simulink model "WMR_ROS_MATMPC_SIMULINK_real"  (R2022b)
settings: Solver=FixedStepAuto  StartTime=0.0  StopTime=100  FixedStep=0.02  RelTol=1e-3
model workspace (MAT data in the model file):
  SL_ROS_VariableLengthArrays_MaxSizes.CommonInfo.ArrayTruncateAction = 'EmitWarning'
  SL_ROS_VariableLengthArrays_MaxSizes.MsgTypeMap = containers.Map
  SL_ROS_VariableLengthArrays_MaxSizes.MsgTypeMap.serialization.keys = {'nav_msgs/OccupancyGrid'}
  SL_ROS_VariableLengthArrays_MaxSizes.MsgTypeMap.serialization.values{1}.PropertyName = 'Data'
  SL_ROS_VariableLengthArrays_MaxSizes.MsgTypeMap.serialization.values{1}.DataType = 'int8'
  SL_ROS_VariableLengthArrays_MaxSizes.MsgTypeMap.serialization.values{1}.MaxLength = 40000
  SL_ROS_VariableLengthArrays_MaxSizes.MsgTypeMap.serialization.uniformity = 0
  SL_ROS_VariableLengthArrays_MaxSizes.MsgTypeMap.serialization.keyType = 'char'
  SL_ROS_VariableLengthArrays_MaxSizes.MsgTypeMap.serialization.valueType = 'any'
values from neighbouring files (symbols this model uses):
  costmap_resolution = 0.1    [Initialization_Simulink.m]
  costmap_width = 100    [Initialization_Simulink.m]
  lb = 0    [Initialization_Simulink.m]
  lb_x = [0;0]    [InitData.m]    (also in Initialization_Simulink.m = [0; -0.8])
  lbu = -inf(nu,1)    [InitData.m]    (also in Initialization_Simulink.m = repmat(lbu,1,N))
  lbx = 0    [Initialization_Simulink.m]
  N = settings.N    [InitData.m]    (also in InitMemory.m; Initialization_Simulink.m = 100; Simulation.m = 10)
  np = settings.np    [InitData.m]    (also in InitMemory.m; Initialization_Simulink.m; Simulation.m)
  Ts = settings.Ts_st    [Initialization_Simulink.m]    (also in Simulation.m)
  ub = 0    [Initialization_Simulink.m]
  ub_x = [100;100]    [InitData.m]    (also in Initialization_Simulink.m = [0.3; 0.8])
  ubu = inf(nu,1)    [InitData.m]    (also in Initialization_Simulink.m = repmat(ubu,1,N))
  ubx = 0    [Initialization_Simulink.m]
  W = repmat(w,1,N)    [Initialization_Simulink.m]
  WN = [50 50 0 50 50]'    [Initialization_Simulink.m]
  z0 = 0    [Initialization_Simulink.m]
undefined symbols (not defined in the file or in its folder): Angular, DiscIntNeverNeededParam, Linear, myref, opt, settings, X, X_SL_Info, Y, Y_SL_Info
libraries: robotlib x8, robotcorelib x2
settings Model: SimulationMode=accelerator  Creator=chen  LastModifiedBy=niccoloturcato
settings SolverCC: AlgebraicLoopSolver=TrustRegion
settings DataIOCC: SaveFormat=StructureWithTime
settings OptimizationCC: EnhancedBackFolding=on  PassReuseOutputArgsAs=Individual arguments  ZeroExternalMemoryAtStartup=off  ZeroInternalMemoryAtStartup=off  MaxStackSize=64  OptimizeBlockOrder=speed  DifferentSizesBufferReuse=on  OptimizationCustomize=off  EfficientTunableParamExpr=on
settings DebuggingCC: ParameterTunabilityLossMsg=error  UnconnectedInputMsg=warning  UnconnectedOutputMsg=warning  UnconnectedLineMsg=warning  SFMachineParentedDataDiag=warning  ArithmeticOperatorsInVariantConditions=warning
settings HardwareCC: ProdBitPerPointer=32  ProdBitPerSizeT=32  ProdBitPerPtrDiffT=32  ProdLargestAtomicFloat=None  ProdIntDivRoundTo=Undefined  ProdEndianess=Unspecified  ProdWordSize=32  ProdHWDeviceType=Generic->Unspecified (assume 32-bit Generic)  UseEmbeddedCoderFeatures=off
settings ModelReferenceCC: EnableRefExpFcnMdlSchedulingChecks=on
settings SFSimCC: SimUseLocalCustomCode=off  MATLABDynamicMemAlloc=off  CustomCodeUndefinedFunction=UseInterfaceOnly
settings RTWCC: Description=Embedded Coder  SystemTargetFile=ert.tlc  HardwareBoard=Robot Operating System (ROS)  TLCOptions="-aInlineSetEventsForThisBaseRateFcn=TLC_FALSE -aSuppressMultiTaskScheduler=TLC_FALSE  -aRateBasedStepFcn=0"  TemplateMakefile=ert_default_tmf  RTWUseLocalCustomCode=off  Toolchain=Catkin  TargetLang=C++  CheckMdlBeforeBuild=Error
settings CodeAppCC: ForceParamTrailComments=on  IgnoreCustomStorageClasses=off  OperatorAnnotations=on  SimulinkDataObjDesc=on  SFDataObjDesc=on  InsertBlockDesc=on
settings ERTTargetCC: SupportNonInlinedSFcns=on

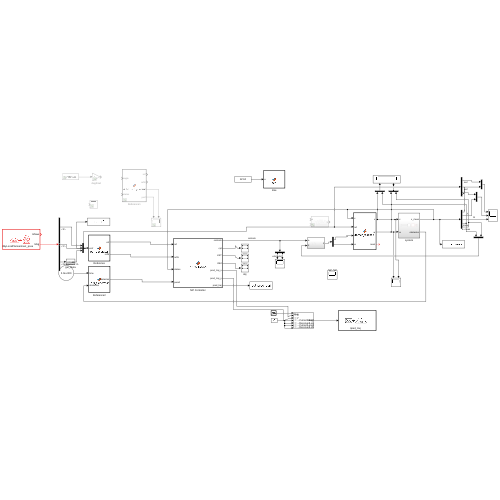
[thumbnail: Simulink's stored preview of the top-level diagram]
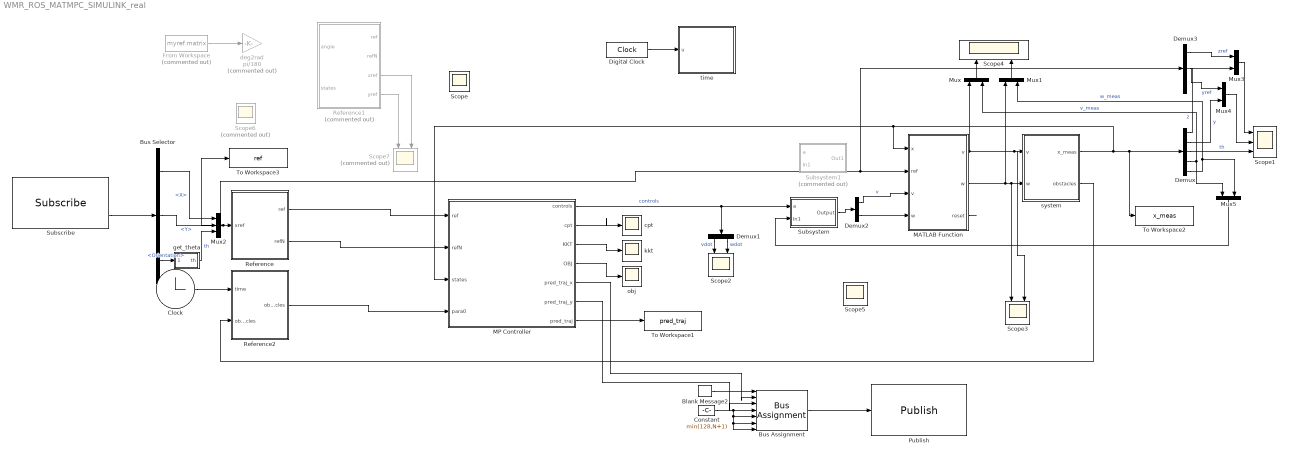
== system WMR_ROS_MATMPC_SIMULINK_real ==
  Blank Message2 : robotlib/Blank Message  messageClass=Message  entityType=wheelchair_iaslab_control/matArray  messageType=wheelchair_iaslab_control/matArray  SampleTime=-1  legacyBusStruct=off
  Bus Assignment : BusAssignment  AssignedSignals=X,Y,X_SL_Info.CurrentLength,X_SL_Info.ReceivedLength,Y_SL_Info.CurrentLength,Y_SL_Info.ReceivedLength
  Bus Selector : BusSelector  DialogController=Simulink.DDGSource_BusSelector  OutputSignals=Position.X,Position.Y,Orientation
  Clock : Clock
  Constant : Constant  Value=min(128,N+1)  OutDataTypeStr=uint32
  Demux : Demux  Outputs=5
  Demux1 : Demux  Outputs=2
  Demux2 : Demux  Outputs=2
  Demux3 : Demux  Outputs=3
  Digital Clock : DigitalClock  SampleTime=-1
  From Workspace : FromWorkspace  Commented=on  VariableName=myref.matrix  SampleTime=myref.T
  MATLAB Function : MATLAB Function  TreatAsAtomicUnit=on
  MP Controller : MATLAB Function  TreatAsAtomicUnit=on  SystemSampleTime=Ts
  Mux{,1,3..5} (5 alike) : Mux  Inputs=2
  Mux2 : Mux  Inputs=3
  Publish : robotlib/Publish  topicSource=Specify your own  topic=/pred_traj  messageType=wheelchair_iaslab_control/matArray  legacyBusStruct=off  messageQueueLength=1
      settings: LibrarySourceBlock=roslib/ROS/Publish
  Reference : MATLAB Function  TreatAsAtomicUnit=on
  Reference1 : MATLAB Function  Commented=on  TreatAsAtomicUnit=on
  Reference2 : MATLAB Function  TreatAsAtomicUnit=on
  Scope1 : Scope  NumInputPorts=3
  Scope{2..5} (4 alike) : Scope  NumInputPorts=2
  Scope6 : Scope  Commented=on
  Scope7 : Scope  Commented=on  NumInputPorts=2
  Subscribe : robotlib/Subscribe  topicSource=Specify your own  topic=/move_base/MyLocalPlanner/next_pose  messageType=geometry_msgs/Pose  SampleTime=0.2  legacyBusStruct=off  messageQueueLength=1
      settings: LibrarySourceBlock=roslib/ROS/Subscribe
  Subsystem : Subsystem
  Subsystem1 : Subsystem  Commented=on
  To Workspace1 : ToWorkspace  VariableName=pred_traj  SaveFormat=Structure With Time  SampleTime=-1
  To Workspace2 : ToWorkspace  VariableName=x_meas  SaveFormat=Structure With Time  SampleTime=-1
  To Workspace3 : ToWorkspace  VariableName=ref  SaveFormat=Structure With Time  SampleTime=-1
  cpt : Scope
  deg2rad : Gain  Commented=on  Gain=pi/180
  get_theta : Subsystem
  kkt : Scope
  obj : Scope
  system : Subsystem
  time : MATLAB Function  TreatAsAtomicUnit=on  SystemSampleTime=Ts
  Scope : Scope
  wires:
  MP Controller/1(controls) -> Subsystem/1(a), Demux1/1  "controls"
  MP Controller/2(cpt) -> cpt/1
  MP Controller/4(OBJ) -> obj/1
  MP Controller/3(KKT) -> kkt/1
  Demux/3 -> Scope1/3  "th"
  Demux/1 -> Mux3/2  "z"
  Demux/2 -> Mux4/2  "y"
  Demux/5 -> Mux5/2, Mux1/2  "w_meas"
  Demux/4 -> Mux/2, Mux5/1  "v_meas"
  Demux1/1 -> Scope2/1  "vdot"
  Demux1/2 -> Scope2/2  "wdot"
  Mux/1 -> Scope4/1
  Mux1/1 -> Scope4/2
  Blank Message2/1 -> Bus Assignment/1
  Bus Assignment/1 -> Publish/1
  MP Controller/6(pred_traj_y) -> Bus Assignment/3
  Constant/1 -> Bus Assignment/7, Bus Assignment/6, Bus Assignment/5, Bus Assignment/4
  Reference/1(ref) -> MP Controller/1(ref)
  Reference/2(refN) -> MP Controller/2(refN)
  From Workspace/1 -> deg2rad/1
  Reference1/3(zref) -> Scope7/2
  Reference1/4(yref) -> Scope7/1
  Clock/1 -> Reference2/1(time)
  Reference2/1(obstacles) -> MP Controller/4(para0)
  system/2(obstacles) -> Reference2/2("obstacles ")
  system/1(x_meas) -> To Workspace2/1, Demux/1, MP Controller/3(states), MATLAB Function/1(x)
  Subscribe/2 -> Bus Selector/1
  Bus Selector/1 -> Mux2/1  "<X>"
  Bus Selector/2 -> Mux2/2  "<Y>"
  Mux2/1 -> To Workspace3/1, Demux3/1, MATLAB Function/2(ref), Reference/1(xref)
  Demux2/1 -> MATLAB Function/3("v ")  "v"
  MATLAB Function/1(v) -> Scope3/2, system/1(v), Mux/1
  MATLAB Function/2(w) -> Scope3/1, system/2(w), Mux1/1
  MATLAB Function/3(reset) -> ?
  Demux3/1 -> Mux3/1  "zref"
  Mux3/1 -> Scope1/1
  Demux3/2 -> Mux4/1  "yref"
  Mux4/1 -> Scope1/2
  MP Controller/5(pred_traj_x) -> Bus Assignment/2
  MP Controller/7(pred_traj) -> To Workspace1/1
  Digital Clock/1 -> time/1(u)
  Bus Selector/3 -> get_theta/1(<Orientation>)  "<Orientation>"
  get_theta/1(th) -> Mux2/3  "th"
  Mux5/1 -> Subsystem/2(In1)
  Demux2/2 -> MATLAB Function/4("w ")
  Subsystem/1(Output) -> Demux2/1

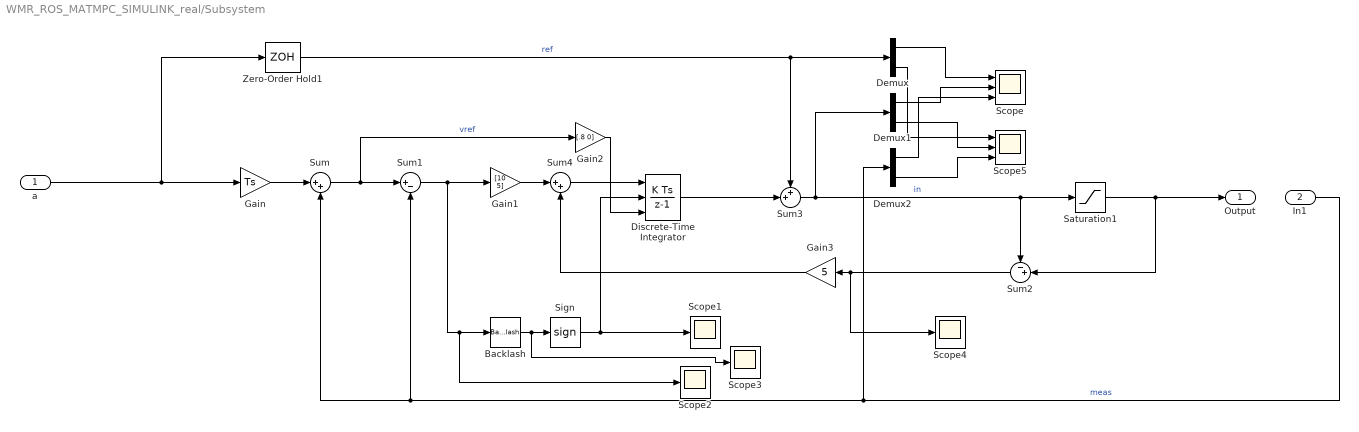
== system WMR_ROS_MATMPC_SIMULINK_real/Subsystem ==
  a : Inport
  In1 : Inport  Port=2
  Backlash : Backlash  BacklashWidth=0.01
  Demux : Demux  Outputs=2
  Demux1 : Demux  Outputs=2
  Demux2 : Demux  Outputs=2
  Discrete-Time Integrator : DiscreteIntegrator  ExternalReset=either  InitialConditionSource=external  SampleTime=-1  ICPrevOutput=DiscIntNeverNeededParam  ICPrevScaledInput=DiscIntNeverNeededParam
  Gain : Gain  Gain=Ts
  Gain1 : Gain  Gain=[10 5]
  Gain2 : Gain  Gain=[.8 0]
  Gain3 : Gain  Gain=5
  Saturation1 : Saturate  UpperLimit=ub_x  LowerLimit=[-0.1 lbx(2)]
  Scope : Scope  NumInputPorts=3
  Scope{1..4} (4 alike) : Scope
  Scope5 : Scope  NumInputPorts=3
  Sign : Signum
  Sum : Sum  Inputs=|++
  Sum1 : Sum  Inputs=|+-
  Sum2 : Sum  Inputs=-+|
  Sum3 : Sum  Inputs=++|
  Sum4 : Sum  Inputs=|++
  Zero-Order Hold1 : ZeroOrderHold  SampleTime=0.02
  Output : Outport
  wires:
  Gain/1 -> Sum/1
  Sum/1 -> Gain2/1, Sum1/1  "vref"
  Backlash/1 -> Scope3/1, Sign/1
  In1/1 -> Sum1/2, Sum/2, Demux2/1  "meas"
  Sum1/1 -> Scope2/1, Backlash/1, Gain1/1
  a/1 -> Zero-Order Hold1/1, Gain/1
  Zero-Order Hold1/1 -> Sum3/1, Demux/1  "ref"
  Discrete-Time Integrator/1 -> Sum3/2
  Sign/1 -> Scope1/1, Discrete-Time Integrator/2
  Gain2/1 -> Discrete-Time Integrator/3
  Sum3/1 -> Demux1/1, Saturation1/1, Sum2/1  "in"
  Saturation1/1 -> Output/1, Sum2/2
  Gain1/1 -> Sum4/1
  Sum4/1 -> Discrete-Time Integrator/1
  Gain3/1 -> Sum4/2
  Sum2/1 -> Scope4/1, Gain3/1
  Demux1/1 -> Scope/2
  Demux2/1 -> Scope/3
  Demux/1 -> Scope/1
  Demux/2 -> Scope5/1
  Demux1/2 -> Scope5/2
  Demux2/2 -> Scope5/3

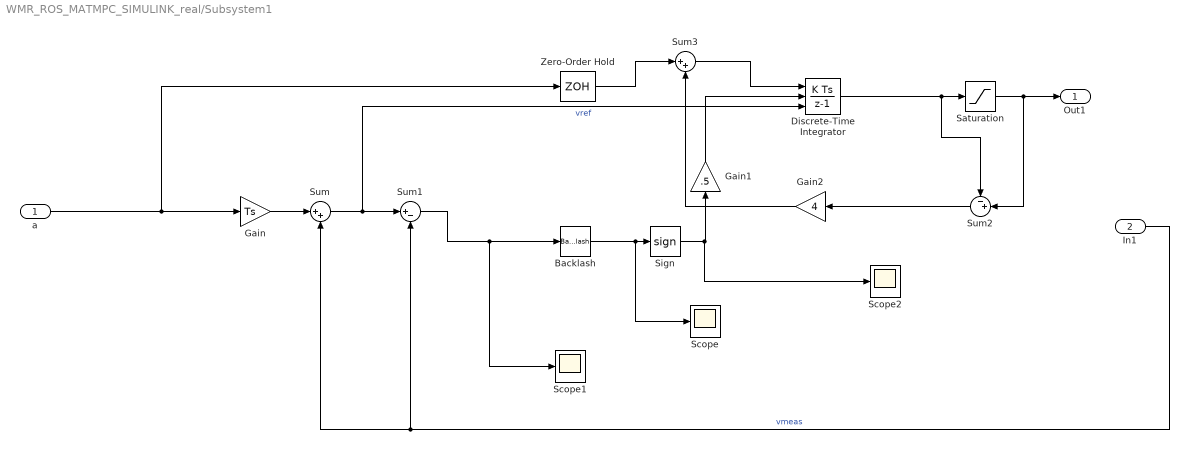
== system WMR_ROS_MATMPC_SIMULINK_real/Subsystem1 ==
  a : Inport
  In1 : Inport  Port=2
  Backlash : Backlash  BacklashWidth=0.01
  Discrete-Time Integrator : DiscreteIntegrator  ExternalReset=either  InitialConditionSource=external  SampleTime=-1  ICPrevOutput=DiscIntNeverNeededParam  ICPrevScaledInput=DiscIntNeverNeededParam
  Gain : Gain  Gain=Ts
  Gain1 : Gain  Gain=.5
  Gain2 : Gain  Gain=4
  Saturation : Saturate  UpperLimit=ub_x  LowerLimit=[-0.1 lbx(2)]
  Scope : Scope
  Scope1 : Scope
  Scope2 : Scope
  Sign : Signum
  Sum : Sum  Inputs=|++
  Sum1 : Sum  Inputs=|+-
  Sum2 : Sum  Inputs=-+|
  Sum3 : Sum  Inputs=|++
  Zero-Order Hold : ZeroOrderHold  SampleTime=0.02
  Out1 : Outport
  wires:
  Gain/1 -> Sum/1
  Sum/1 -> Discrete-Time Integrator/3, Sum1/1  "vref"
  Backlash/1 -> Scope/1, Sign/1
  In1/1 -> Sum1/2, Sum/2  "vmeas"
  Sum1/1 -> Scope1/1, Backlash/1
  Sign/1 -> Gain1/1, Scope2/1
  Discrete-Time Integrator/1 -> Sum2/1, Saturation/1
  Gain1/1 -> Discrete-Time Integrator/2
  Saturation/1 -> Sum2/2, Out1/1
  a/1 -> Zero-Order Hold/1, Gain/1
  Zero-Order Hold/1 -> Sum3/1
  Sum2/1 -> Gain2/1
  Gain2/1 -> Sum3/2
  Sum3/1 -> Discrete-Time Integrator/1

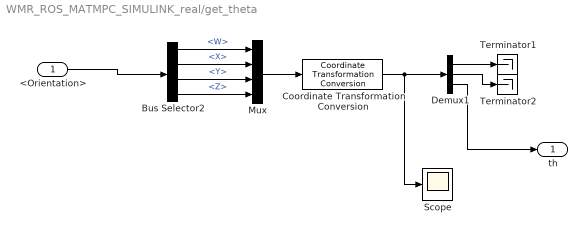
== system WMR_ROS_MATMPC_SIMULINK_real/get_theta ==
  <Orientation> : Inport
  Bus Selector2 : BusSelector  DialogController=Simulink.DDGSource_BusSelector  OutputSignals=W,X,Y,Z
  Coordinate Transformation Conversion : robotcorelib/Coordinate Transformation Conversion  InputRepresentation=Quaternion  InputEulerSequence=ZYX  ShowTrVecInputPort=on  OutputRepresentation=Euler Angles  OutputEulerSequence=XYZ  ShowTrVecOutputPort=on  SimulateUsing=Interpreted execution
      settings: LibrarySourceBlock=roslib/Utilities/Coordinate Transformation Conversion
  Demux1 : Demux  Outputs=3
  Mux : Mux
  Scope : Scope
  Terminator1 : Terminator
  Terminator2 : Terminator
  th : Outport
  wires:
  Bus Selector2/3 -> Mux/3  "<Y>"
  Demux1/1 -> Terminator1/1
  Bus Selector2/4 -> Mux/4  "<Z>"
  Bus Selector2/1 -> Mux/1  "<W>"
  Coordinate Transformation Conversion/1 -> Scope/1, Demux1/1
  <Orientation>/1 -> Bus Selector2/1
  Demux1/2 -> Terminator2/1
  Bus Selector2/2 -> Mux/2  "<X>"
  Mux/1 -> Coordinate Transformation Conversion/1
  Demux1/3 -> th/1

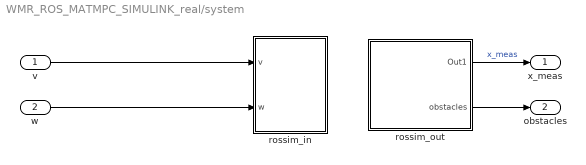
== system WMR_ROS_MATMPC_SIMULINK_real/system ==
  v : Inport
  w : Inport  Port=2
  rossim_in : Subsystem
  rossim_out : Subsystem
  x_meas : Outport
  obstacles : Outport  Port=2
  wires:
  w/1 -> rossim_in/2(w)
  v/1 -> rossim_in/1(v)
  rossim_out/1(Out1) -> x_meas/1  "x_meas"
  rossim_out/2(obstacles) -> obstacles/1

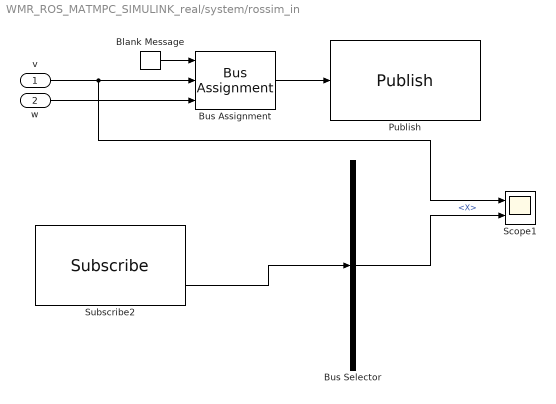
== system WMR_ROS_MATMPC_SIMULINK_real/system/rossim_in ==
  v : Inport
  w : Inport  Port=2
  Blank Message : robotlib/Blank Message  messageClass=Message  entityType=geometry_msgs/Twist  messageType=geometry_msgs/Twist  SampleTime=-1  legacyBusStruct=off
  Bus Assignment : BusAssignment  AssignedSignals=Linear.X,Angular.Z
  Bus Selector : BusSelector  DialogController=Simulink.DDGSource_BusSelector  OutputSignals=Linear.X
  Publish : robotlib/Publish  topicSource=Specify your own  topic=/cmd_vel  messageType=geometry_msgs/Twist  legacyBusStruct=off  messageQueueLength=1
      settings: LibrarySourceBlock=roslib/ROS/Publish
  Scope1 : Scope  NumInputPorts=2
  Subscribe2 : robotlib/Subscribe  topicSource=Specify your own  topic=/cmd_vel  messageType=geometry_msgs/Twist  SampleTime=0.020  legacyBusStruct=off  messageQueueLength=1
      settings: LibrarySourceBlock=roslib/ROS/Subscribe
  wires:
  Blank Message/1 -> Bus Assignment/1
  Bus Assignment/1 -> Publish/1
  v/1 -> Scope1/1, Bus Assignment/2
  Subscribe2/2 -> Bus Selector/1
  Bus Selector/1 -> Scope1/2  "<X>"
  w/1 -> Bus Assignment/3

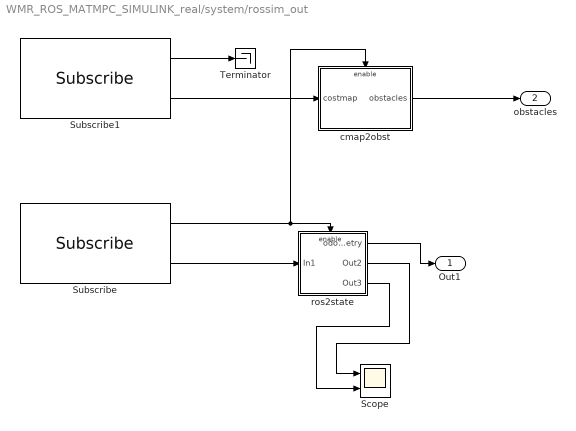
== system WMR_ROS_MATMPC_SIMULINK_real/system/rossim_out ==
  Scope : Scope  NumInputPorts=2
  Subscribe : robotlib/Subscribe  topicSource=Specify your own  topic=/odom  messageType=nav_msgs/Odometry  SampleTime=0.020  legacyBusStruct=off  messageQueueLength=1
      settings: LibrarySourceBlock=roslib/ROS/Subscribe
  Subscribe1 : robotlib/Subscribe  topicSource=Select from ROS network  topic=/move_base/local_costmap/costmap  messageType=nav_msgs/OccupancyGrid  SampleTime=0.02  legacyBusStruct=off  messageQueueLength=1
      settings: LibrarySourceBlock=roslib/ROS/Subscribe
  Terminator : Terminator
  cmap2obst : Subsystem
  ros2state : Subsystem
  Out1 : Outport
  obstacles : Outport  Port=2
  wires:
  Subscribe/1 -> ros2state/Enable, cmap2obst/Enable
  Subscribe/2 -> ros2state/1(In1)
  ros2state/1(odometry) -> Out1/1
  ros2state/2(Out2) -> Scope/1
  ros2state/3(Out3) -> Scope/2
  Subscribe1/1 -> Terminator/1
  Subscribe1/2 -> cmap2obst/1(costmap)
  cmap2obst/1(obstacles) -> obstacles/1

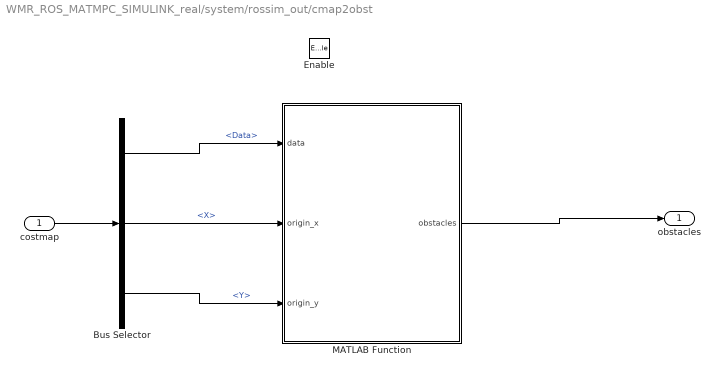
== system WMR_ROS_MATMPC_SIMULINK_real/system/rossim_out/cmap2obst ==
  costmap : Inport
  Enable : EnablePort  StatesWhenEnabling=reset
  Bus Selector : BusSelector  DialogController=Simulink.DDGSource_BusSelector  OutputSignals=Data,Info.Origin.Position.X,Info.Origin.Position.Y
  MATLAB Function : MATLAB Function  TreatAsAtomicUnit=on
  obstacles : Outport
  wires:
  costmap/1 -> Bus Selector/1
  MATLAB Function/1(obstacles) -> obstacles/1
  Bus Selector/3 -> MATLAB Function/3(origin_y)  "<Y>"
  Bus Selector/2 -> MATLAB Function/2(origin_x)  "<X>"
  Bus Selector/1 -> MATLAB Function/1(data)  "<Data>"

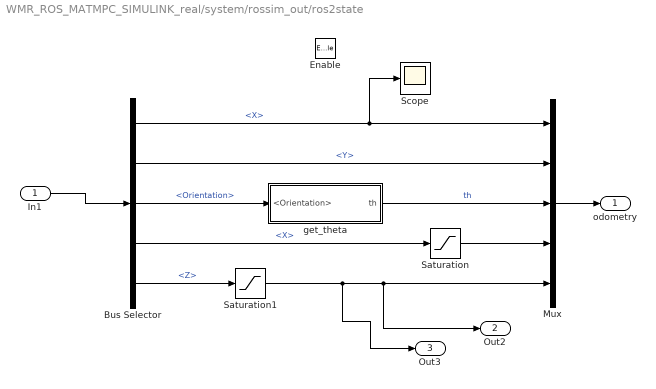
== system WMR_ROS_MATMPC_SIMULINK_real/system/rossim_out/ros2state ==
  In1 : Inport
  Enable : EnablePort  StatesWhenEnabling=reset
  Bus Selector : BusSelector  DialogController=Simulink.DDGSource_BusSelector  OutputSignals=Pose.Pose.Position.X,Pose.Pose.Position.Y,Pose.Pose.Orientation,Twist.Twist.Linear.X,Twist.Twist.Angular.Z
  Mux : Mux  Inputs=5
  Saturation : Saturate  UpperLimit=ub_x(1)  LowerLimit=lb_x(1)
  Saturation1 : Saturate  UpperLimit=ub_x(2)  LowerLimit=lb_x(2)
  Scope : Scope
  get_theta : Subsystem
  odometry : Outport
  Out2 : Outport  Port=2
  Out3 : Outport  Port=3
  wires:
  Bus Selector/5 -> Saturation1/1  "<Z>"
  Bus Selector/1 -> Mux/1, Scope/1  "<X>"
  In1/1 -> Bus Selector/1
  get_theta/1(th) -> Mux/3  "th"
  Bus Selector/2 -> Mux/2  "<Y>"
  Bus Selector/3 -> get_theta/1(<Orientation>)  "<Orientation>"
  Bus Selector/4 -> Saturation/1  "<X>"
  Mux/1 -> odometry/1
  Saturation/1 -> Mux/4
  Saturation1/1 -> Mux/5, Out2/1, Out3/1

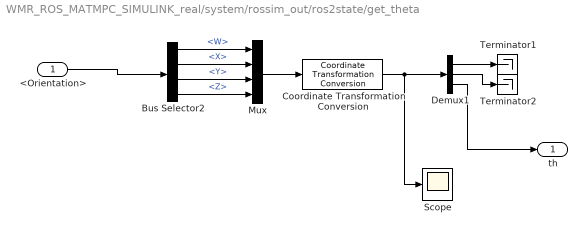
== system WMR_ROS_MATMPC_SIMULINK_real/system/rossim_out/ros2state/get_theta ==
  <Orientation> : Inport
  Bus Selector2 : BusSelector  DialogController=Simulink.DDGSource_BusSelector  OutputSignals=W,X,Y,Z
  Coordinate Transformation Conversion : robotcorelib/Coordinate Transformation Conversion  InputRepresentation=Quaternion  InputEulerSequence=ZYX  ShowTrVecInputPort=on  OutputRepresentation=Euler Angles  OutputEulerSequence=XYZ  ShowTrVecOutputPort=on  SimulateUsing=Interpreted execution
      settings: LibrarySourceBlock=roslib/Utilities/Coordinate Transformation Conversion
  Demux1 : Demux  Outputs=3
  Mux : Mux
  Scope : Scope
  Terminator1 : Terminator
  Terminator2 : Terminator
  th : Outport
  wires:
  Bus Selector2/3 -> Mux/3  "<Y>"
  Demux1/1 -> Terminator1/1
  Bus Selector2/4 -> Mux/4  "<Z>"
  Bus Selector2/1 -> Mux/1  "<W>"
  Coordinate Transformation Conversion/1 -> Scope/1, Demux1/1
  <Orientation>/1 -> Bus Selector2/1
  Demux1/2 -> Terminator2/1
  Bus Selector2/2 -> Mux/2  "<X>"
  Mux/1 -> Coordinate Transformation Conversion/1
  Demux1/3 -> th/1

== matlab function WMR_ROS_MATMPC_SIMULINK_real/MP Controller ==
  settings: updateMethod=DISCRETE  sampleTime=Ts
  data: settings parameter; opt parameter; lb parameter; ub parameter; lbx parameter; ubx parameter; lbu parameter; ubu parameter; W parameter; WN parameter; ref input size=[ny N]; refN input size=nyN; z0 parameter; states input size=nx; N parameter; controls output size=nu; cpt output size=1; KKT output; OBJ output; pred_traj_x output; pred_traj_y output; para0 input; pred_traj output
function [controls, cpt, KKT, OBJ,pred_traj_x,pred_traj_y,pred_traj]  = NMPC_BLOCK(settings, opt, lb, ub, lbx, ubx, lbu, ubu, W, WN, ref, refN, z0, states,N, para0)

%% everything should have a fixed size
coder.extrinsic('mpc_nmpcsolver_simulink');  
coder.extrinsic('InitData');  
coder.extrinsic('InitMemory');  
coder.extrinsic('evalin');
coder.extrinsic('assignin');

%%

persistent x u z lambda mu mu_x mu_u;
persistent input mem;

%% !!DAVIDE TEST!!
%     obstacles = 2*zeros(10,1);
%     obstacles(1)=3;
%     obstacles(2)=0;
    para = repmat(para0,1,settings.N+1);

%%

if isempty(input)  
    
    nx = settings.nx;        % No. of differential states
    nu = settings.nu;        % No. of controls
    nz = settings.nz;        % No. of algebraic states
    ny = settings.ny;        % No. of outputs (references)    
    nyN= settings.nyN;       % No. of outputs at terminal stage 
    np = settings.np;        % No. of parameters (on-line data)
    nc = settings.nc;        % No. of constraints
    ncN = settings.ncN;      % No. of constraints at terminal stage
    nbu = settings.nbu;      % No. of control bounds
    nbx = settings.nbx;      % No. of state bounds
    nbu_idx = settings.nbu_idx; % Index of control bounds
    nbx_idx = settings.nbx_idx; % Index of state bounds
    N = settings.N;
    N2 = settings.N2;
    r = settings.r;
        
    input.x0=states;
    
    x=repmat(states,1,N+1);
    input.x=x;
    
    u=zeros(nu,N);
    input.u=u;
    
    z=repmat(z0,1,N);
    input.z=z;
    
    lambda = zeros(nx,N+1);
    input.lambda= lambda;
    
    if N*nc+ncN > 0
        mu = zeros(N*nc+ncN,1);
    else
        mu = 0;
    end
    input.mu= mu;
    
    mu_u = zeros(N*nu,1);
    input.mu_u= mu_u;
    
    if N*nbx > 0
        mu_x = zeros(N*nbx,1);
    else
        mu_x = 0;
    end
    input.mu_x = mu_x;
    
    input.W=W;
    input.WN=WN;
    input.od = para;
    
    input.lb = lb;
    input.ub = ub;
    input.lbx = lbx;
    input.ubx = ubx;
    input.lbu = lbu;
    input.ubu = ubu;
      
    input.y = ref;
    input.yN = refN;
    
    mem = InitMemory(settings, opt, input);
        
else

    input.x=x; 
    input.u=u;
    input.z=z;
    input.lambda=lambda;   
    input.mu=mu;
    input.mu_x=mu_x;
    input.mu_u=mu_u;
    input.od = para;
    input.y = ref;
    input.yN = refN;
    
end

%%
cpt = 0;
KKT = 0;
OBJ = 0;
input.x0 = states;

%%DAVIDE
pred_traj_x = zeros(128,1);
pred_traj_y = zeros(128,1);

pred_traj_x(1:min(N+1,128)) = input.x(1,1:min(128,N+1))';
pred_traj_y(1:min(N+1,128)) = input.x(2,1:min(128,N+1))';

pred_traj = [pred_traj_x,pred_traj_y];

[input,mem,cpt,KKT,OBJ] = mpc_nmpcsolver_simulink(input, settings, mem, opt);
controls = input.u(:,1);

%% shifting
switch opt.shifting
    case 'yes'
        x=[input.x(:,2:end),input.x(:,end)];  
        u=[input.u(:,2:end),input.u(:,end)]; 
        z=[input.z(:,2:end),input.z(:,end)]; 
        lambda=[input.lambda(:,2:end),input.lambda(:,end)];
        if (settings.N*settings.nc+settings.ncN) >0
            mu(1:end-settings.ncN+1)=input.mu(settings.nc+1:settings.N*settings.nc+settings.ncN,1);
            mu(settings.N*settings.nc+1:end)=input.mu(settings.N*settings.nc+settings.ncN-settings.nc+1:settings.N*settings.nc+settings.ncN,1);
        else
            mu=0;
        end
        mu_x=[input.mu_x(2:end,1);input.mu_x(end,1)];
        mu_u=[input.mu_u(2:end,1);input.mu_u(end,1)];
   case 'no'
        x=input.x;
        u=input.u;
        z=input.z;
        lambda=input.lambda;
        mu=input.mu;
        mu_x=input.mu_x;
        mu_u=input.mu_u;
end

return

== matlab function WMR_ROS_MATMPC_SIMULINK_real/Reference ==
  data: ref output; settings parameter; refN output; xref input
function [ref,refN] = Ref_Generator(settings, xref)
        
%     persistent zref yref count;

%     x_meas = zeros(5,1);

%     references = [[1,0];[2,-1];[2,-2];[3,-3];[5,-3]];
    %references = [[2,-1];[3,-3];[5,-3]];

%     zref = 2;
%     yref = 0;

    zref = xref(1);
    yref = xref(2);
    thref = xref(3);

%     if isempty(zref)
%         count = 1;
%         zref = references(1,1);
%         yref = references(1,2);
%         disp(zref)
%         disp(yref)
%     else
%     
%         zwc = x_meas(1);
%         ywc = x_meas(2);
%     
%         dist = sqrt((zref-zwc)^2 + (yref-ywc)^2);
%     
%         if dist < 0.25 && count<=length(references)
%             count = count+1;
%             zref = references(count,1);
%             yref = references(count,2);
%             disp('switch!')
%             disp(zref)
%             disp(yref)
%         end
%        
%     end
    
    ref = repmat([zref,yref,thref,0,0,0,0]',1,settings.N);
    refN = [zref,yref,thref,0,0]';

end

== matlab function WMR_ROS_MATMPC_SIMULINK_real/system/rossim_out/cmap2obst/MATLAB Function ==
  data: obstacles output size=np; data input; origin_x input; origin_y input; costmap_resolution parameter; costmap_width parameter; np parameter
function obstacles = costmap2obstacles(data, origin_x, origin_y, costmap_resolution, costmap_width, np)
% obstacles_num is the number of obstacles
% obstacles_pos is 1 x np=len
% obstacles_pos = (obstacles_num, px1,py1,px2,py2,...,0,0,0,0)

obstacles = zeros(np,1);
% for i = 1 : 2 : length(obstacles)
%     obstacles(i) = 3;
% end


count = 0; 
no = 1000;
all_obstacles_ij = zeros(no,2);
all_obstacles_priorities = zeros(no,1);

for i = 1 : costmap_width^2
    iy = ceil(i/costmap_width);
    ix = i - (iy-1)*costmap_width;
    if data(i)>=100 && count<=no
        count = count+1;
        all_obstacles_ij(count,:) = [ix,iy];
        priority = - (ix-costmap_width/2)^2 - (iy-costmap_width/2)^2;
        all_obstacles_priorities(count) = priority;
    end
end

if count == 0
    disp('No obstaces!')
else
    [~,idx] = sort(all_obstacles_priorities(1:count));
    
    for i = 1 : np/2
        if i<=count
            j = idx(i);
            point = all_obstacles_ij(j,:);
            ix = point(1);
            iy = point(2);
            px = (ix-0.5)*costmap_resolution + origin_x;
            py = (iy-0.5)*costmap_resolution + origin_y;
            obstacles(2*i-1:2*i) = [px,py];
%             disp([px,py]);
        else
            obstacles(2*i-1:2*i) = obstacles(2*count-1:2*count);
        end
    end
    
%     disp(obstacles)
%  
end

% 
% count = 1; 
% 
% for i = 1 : costmap_width^2
%     iy = ceil(i/costmap_width);
%     ix = i - (iy-1)*costmap_width;
%     if data(i)>99 && count<np
%         px = (ix-0.5)*costmap_resolution + origin_x;
%         py = (iy-0.5)*costmap_resolution + origin_y;
%         obstacles(count:count+1) = [px,py];
%         count = count+2;
%         disp([px,py])
%     end
% end

== matlab function WMR_ROS_MATMPC_SIMULINK_real/Reference2 ==
  data: np parameter; N parameter; obstacles output; time input; obstacles input; Ts parameter
function obstacles  = Para_Generator(np, N, time, obstacles, Ts)

    if time < Ts
        obstacles = -ones(np,1);
%         obstacles(1)=3;
%         obstacles(2)=0;
%         obstacles(3)=3;
%         obstacles(4)=0;
%         obstacles(5)=3;
%         obstacles(6)=0;
%         obstacles(7)=3;
%         obstacles(8)=0;
%         obstacles(9)=3;
%         obstacles(10)=0;
    end
%     obstacles = 2*ones(np,1);
%     obstacles(1)=3;
%     obstacles(2)=0;
    
%     disp(obstacles)

end

== matlab function WMR_ROS_MATMPC_SIMULINK_real/MATLAB Function ==
  data: x input; v output; ref input; v input; w input; w output; reset output
function [v,w, reset] = target_reached(x, ref, v, w)

reset = 0;

z = x(1);
y = x(2);

zref = ref(1);
yref = ref(2);

dist = sqrt((z-zref)^2+(y-yref)^2);

%v = 0;
%w = 0;

if dist<0.4
    v = 0;
    w = 0;
    reset=1;
end

== matlab function WMR_ROS_MATMPC_SIMULINK_real/time ==
  settings: updateMethod=DISCRETE
  data: u input
function fcn(u)
%#codegen
coder.extrinsic('fprintf');
persistent firstTime

if isempty(firstTime)
    firstTime = false;
    fprintf('Starting Now\n');
end
if mod(u,1)==0
    fprintf('time = %.4f\n',u);
end
end

== matlab function WMR_ROS_MATMPC_SIMULINK_real/Reference1 ==
  data: ref output; settings parameter; refN output; myref parameter; angle input; states input; zref output; yref output
function [ref,refN,zref,yref] = variable_ref_generator(settings, myref, angle, states)

    z = states(1);
    y = states(2);
    th = states(3);
    
    zref = z+myref.dist*cos(th+angle);
    yref = y+myref.dist*sin(th+angle);
    
    ref = repmat([zref,yref,0,0,0,0,0]',1,settings.N);
    refN = [zref,yref,0,0,0]';

end
